simulink model "hw5_2"  (R2023a)
settings: Solver=VariableStepAuto  StartTime=0.0  StopTime=15  RelTol=1e-3
libraries: simulink x2
settings Model: Creator=마이컴  LastModifiedBy=마이컴

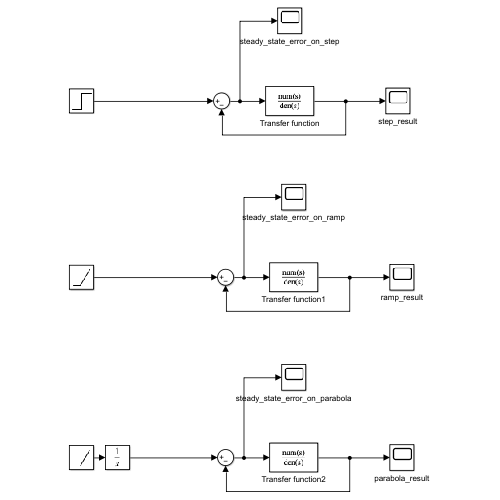
[thumbnail: Simulink's stored preview of the top-level diagram]
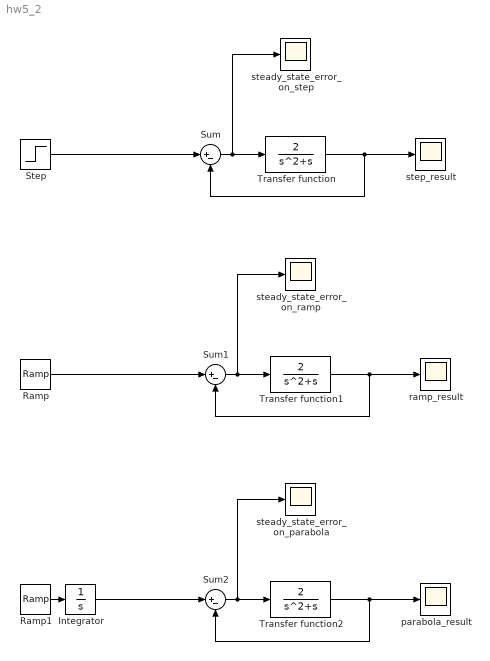
== system hw5_2 ==
  Integrator : Integrator
  Ramp : simulink/Sources/Ramp  slope=1  start=0  InitialOutput=0
  Ramp1 : simulink/Sources/Ramp  slope=1  start=0  InitialOutput=0
  Step : Step  SampleTime=0
  Sum : Sum  Inputs=|+-
  Sum1 : Sum  Inputs=|+-
  Sum2 : Sum  Inputs=|+-
  Transfer function : TransferFcn  Numerator=[2]  Denominator=[1 1 0]
  Transfer function1 : TransferFcn  Numerator=[2]  Denominator=[1 1 0]
  Transfer function2 : TransferFcn  Numerator=[2]  Denominator=[1 1 0]
  parabola_result : Scope
  ramp_result : Scope
  steady_state_error_on_parabola : Scope
  steady_state_error_on_ramp : Scope
  steady_state_error_on_step : Scope
  step_result : Scope
  wires:
  Ramp1/1 -> Integrator/1
  Sum/1 -> steady_state_error_on_step/1, Transfer function/1
  Step/1 -> Sum/1
  Transfer function/1 -> Sum/2, step_result/1
  Transfer function1/1 -> ramp_result/1, Sum1/2
  Ramp/1 -> Sum1/1
  Sum1/1 -> Transfer function1/1, steady_state_error_on_ramp/1
  Sum2/1 -> steady_state_error_on_parabola/1, Transfer function2/1
  Transfer function2/1 -> Sum2/2, parabola_result/1
  Integrator/1 -> Sum2/1
